simulink model "MotorJaulaArdilla3"  (R2022b)
settings: Solver=ode23s  StartTime=0.0  StopTime=10  MaxStep=1e-3  RelTol=1e-3
libraries: spsIGBTDiodeLib x6, simulink x2, spsAsynchronousMachineSIUnitsLib x1, spsDCVoltageSourceLib x1, spsVoltageMeasurementLib x1, sps_lib x1
settings Model: Creator=ONTIBON  LastModifiedBy=ontib

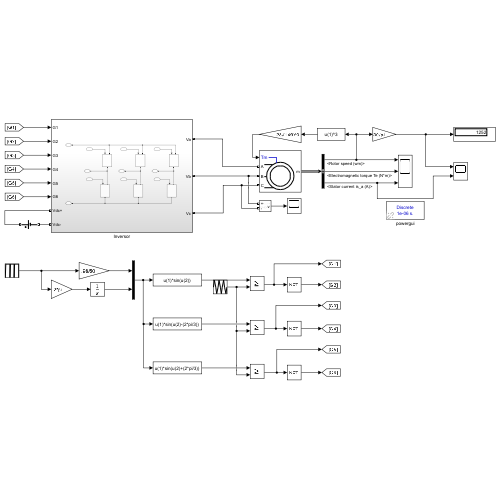
[thumbnail: Simulink's stored preview of the top-level diagram]
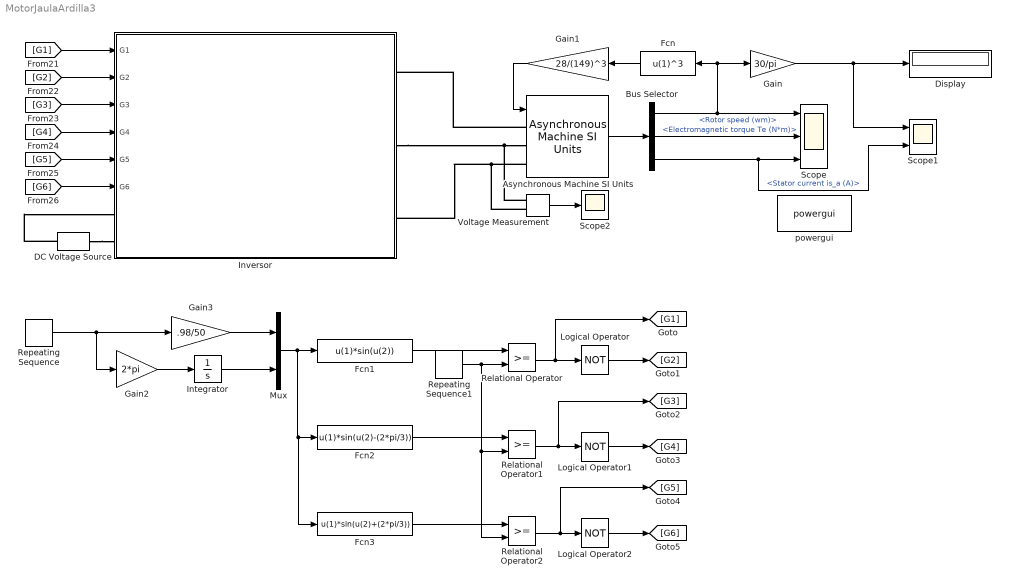
== system MotorJaulaArdilla3 ==
  Asynchronous Machine SI Units : spsAsynchronousMachineSIUnitsLib/Asynchronous Machine SI Units  RotorType=Squirrel-cage  PresetModel="15:  5.4 HP (4KW)   400 V  50Hz 1430 RPM"  MechanicalLoad=Torque Tm  ShowDetailedParameters=on  ReferenceFrame=Rotor  Units=SI  MeasurementBus=off  NominalParameters=[4000 400 50]  VoltageRatio=1  Stator=[1.405 0.005839]  Rotor=[1.395 0.005839]  Cage1=[0.4155 0.002066]  Cage2=[0.4168 0.0003495]  Lm=0.1722  Mechanical=[0.0131 0.002985 2]  PolePairs=2  InitialConditions=[1 0 0 0 0 0 0 0]  SimulateSaturation=off  Saturation=[14.03593122, 27.81365428, 53.79336849, 72.68890987, 97.98006896, 148.6815601, 215.7428561, 302.9841135, 428.7778367 ; 230, 322, 414, 460, 506, 552, 598, 644, 690]  LoadFlowParameters=1492000  TsPowergui=0  TsBlock=-1  IterativeModel=Trapezoidal non iterative  IterativeDiscreteModel=Trapezoidal non iterative  Pmec=1.492e+006
  Bus Selector : BusSelector  OutputSignals=Mechanical.Rotor speed (wm),Mechanical.Electromagnetic torque Te (N*m),Stator measurements.Stator current is_a (A)
  DC Voltage Source : spsDCVoltageSourceLib/DC Voltage Source  Amplitude=650  Measurements=None
  Display : Display
  Fcn : Fcn  Expr=u(1)^3
  Fcn1 : Fcn  Expr=u(1)*sin(u(2))
  Fcn2 : Fcn  Expr=u(1)*sin(u(2)-(2*pi/3))
  Fcn3 : Fcn  Expr=u(1)*sin(u(2)+(2*pi/3))
  Gain : Gain  Gain=30/pi
  Gain1 : Gain  Gain=28/(149)^3
  Gain2 : Gain  Gain=2*pi
  Gain3 : Gain  Gain=.98/50
  Integrator : Integrator
  Inversor : Subsystem
  Logical Operator : Logic  Operator=NOT  AllPortsSameDT=off  OutDataTypeStr=boolean
  Logical Operator1 : Logic  Operator=NOT  AllPortsSameDT=off  OutDataTypeStr=boolean
  Logical Operator2 : Logic  Operator=NOT  AllPortsSameDT=off  OutDataTypeStr=boolean
  Mux : Mux  Inputs=2
  Relational Operator : RelationalOperator  OutDataTypeStr=boolean  RndMeth=Simplest  InputSameDT=off
  Relational Operator1 : RelationalOperator  OutDataTypeStr=boolean  RndMeth=Simplest  InputSameDT=off
  Relational Operator2 : RelationalOperator  OutDataTypeStr=boolean  RndMeth=Simplest  InputSameDT=off
  Repeating Sequence : simulink/Sources/Repeating Sequence  rep_seq_t=[0 1.1 10]  rep_seq_y=[0 50 50]
  Repeating Sequence1 : simulink/Sources/Repeating Sequence  rep_seq_t=[0 .25/5000 .5/5000 .75/5000 1/5000]  rep_seq_y=[0 1 0 -1 0]
  Scope : Scope  NumInputPorts=3
  Scope1 : Scope  NumInputPorts=2
  Scope2 : Scope
  Voltage Measurement : spsVoltageMeasurementLib/Voltage Measurement  PhasorSimulation=off  OutputType=Complex  PSBequivalent=0
  powergui : sps_lib/powergui  Priority=1  SimulationMode=Discrete  SampleTime=1e-6  frequency=60  Iterations=50  frequencyindice=50  Pbase=100e6  ErrMax=1e-4  UnitsV=kV  UnitsW=MW  buscounter=0  FunctionMessages=off  echomessages=off  EnableUseOfTLC=off  CurrentSourceSwitches=off  DisableSnubberDevices=off  DisableRonSwitches=off  DisableVfSwitches=off  DisplayEquations=off  AutomaticDiscreteSolvers=off  SolverType=Tustin/Backward Euler (TBE)  Interpol=off  ExternalGateDelay=off  methode=off  Ts=100  x0status=blocks  SPID=on  SwTol=0  HookPort=off  NonlinearTolerance=1e-4  nMaxIteration=100  ContinueOnMaxIteration=off  RestoreLinks=warning  ResistiveCurrentMeasurement=off  Frange=[0:2:500]  Ylog=off  Xlog=on  ShowGrid=off  save=off  variable=ZData  structure=0  ZoomFFT=off  StartTime=0.0  cycles=1  DisplayStyle=1  fundamental=60  FreqAxis=off  MaxFrequency=1000  frequencyindicesteady=1  RmsSteady=1  display=off
  wires:
  Asynchronous Machine SI Units/1 -> Bus Selector/1
  Gain/1 -> Scope1/1, Display/1
  Bus Selector/1 -> Fcn/1, Gain/1, Scope/1  "<Rotor speed (wm)>"
  Bus Selector/2 -> Scope/2  "<Electromagnetic torque Te (N*m)>"
  Bus Selector/3 -> Scope1/2, Scope/3  "<Stator current is_a (A)>"
  Gain1/1 -> Asynchronous Machine SI Units/1
  Fcn/1 -> Gain1/1
  Mux/1 -> Fcn3/1, Fcn2/1, Fcn1/1
  Integrator/1 -> Mux/2
  Gain2/1 -> Integrator/1
  Gain3/1 -> Mux/1
  Repeating Sequence/1 -> Gain2/1, Gain3/1
  [G2] -> Inversor/2(G2)
  [G1] -> Inversor/1(G1)
  [G4] -> Inversor/4(G4)
  [G6] -> Inversor/6(G6)
  [G3] -> Inversor/3(G3)
  [G5] -> Inversor/5(G5)
  Relational Operator/1 -> [G1], Logical Operator/1
  Fcn1/1 -> Relational Operator/1
  Repeating Sequence1/1 -> Relational Operator2/2, Relational Operator1/2, Relational Operator/2
  Relational Operator1/1 -> [G3], Logical Operator1/1
  Fcn2/1 -> Relational Operator1/1
  Relational Operator2/1 -> [G5], Logical Operator2/1
  Fcn3/1 -> Relational Operator2/1
  Logical Operator/1 -> [G2]
  Logical Operator1/1 -> [G4]
  Logical Operator2/1 -> [G6]
  Voltage Measurement/1 -> Scope2/1
  connections:
  Asynchronous Machine SI Units/LConn1 -- Inversor/RConn1
  DC Voltage Source/LConn1 -- Inversor/LConn2
  Asynchronous Machine SI Units/LConn3 -- Voltage Measurement/LConn2 -- Inversor/RConn3
  Inversor/RConn2 -- Voltage Measurement/LConn1 -- Asynchronous Machine SI Units/LConn2
  DC Voltage Source/RConn1 -- Inversor/LConn1

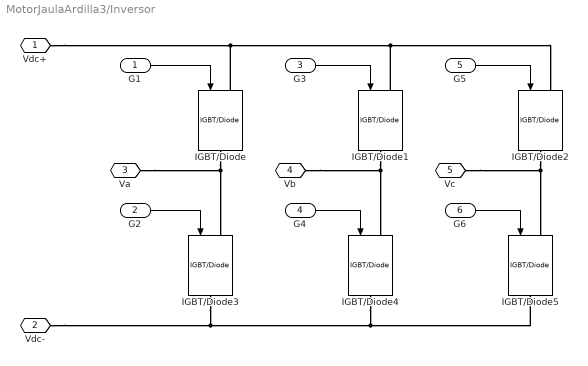
== system MotorJaulaArdilla3/Inversor ==
  G1 : Inport
  G2 : Inport  Port=2
  G3 : Inport  Port=3
  G4 : Inport  Port=4
  G5 : Inport  Port=5
  G6 : Inport  Port=6
  IGBT/Diode{,1..5} (6 alike) : spsIGBTDiodeLib/IGBT//Diode  Ron=1e-3  Rs=1e5  Cs=inf  Measurements=off
  Vdc+ : PMIOPort  Side=Left
  Vdc- : PMIOPort  Port=2  Side=Left
  Va : PMIOPort  Port=3  Side=Right
  Vb : PMIOPort  Port=4  Side=Right
  Vc : PMIOPort  Port=5  Side=Right
  wires:
  G6/1 -> IGBT/Diode5/1
  G1/1 -> IGBT/Diode/1
  G2/1 -> IGBT/Diode3/1
  G3/1 -> IGBT/Diode1/1
  G4/1 -> IGBT/Diode4/1
  G5/1 -> IGBT/Diode2/1
  connections:
  IGBT/Diode2/RConn1 -- Vc/RConn1 -- IGBT/Diode5/LConn1
  IGBT/Diode3/RConn1 -- Vdc-/RConn1 -- IGBT/Diode4/RConn1 -- IGBT/Diode5/RConn1
  IGBT/Diode/RConn1 -- Va/RConn1 -- IGBT/Diode3/LConn1
  IGBT/Diode1/RConn1 -- Vb/RConn1 -- IGBT/Diode4/LConn1
  IGBT/Diode/LConn1 -- Vdc+/RConn1 -- IGBT/Diode1/LConn1 -- IGBT/Diode2/LConn1
